simulink model "BLDC_model"  (R2020a)
settings: Solver=VariableStepAuto  StartTime=0.0  StopTime=10.0  RelTol=1e-3
InitFcn:
  | BLDC_FOC_Params
values from neighbouring files (symbols this model uses):
  AlignmentDuration = 3 * TimeConstant_s    (= 0.2025)    [BLDC_FOC_Params.m]
  AlignmentDuration_s = 1    [BLDC_FOC_Params.m]
  B = FrictionCoefficient_Nms    (= 1e-06)    [BLDC_FOC_Params.m]    (also in BldcModel.m = [1/Ls 0 0 0; systemDynamicsFunction.m = evalin('base','B'))
  J = RotorInertia_KgM2    (= 1.1e-07)    [BLDC_FOC_Params.m]    (also in systemDynamicsFunction.m = evalin('base','J'))
  Ke = BackEmfConstant_VRads    (= 0.00505253787593)    [BLDC_FOC_Params.m]    (also in systemDynamicsFunction.m = evalin('base','Ke'))
  Ls = PhaseSelfInductance_H    (= 0)    [BLDC_FOC_Params.m]    (also in systemDynamicsFunction.m = evalin('base','Ls'))
  MotorPolePairs = 4    [BLDC_FOC_Params.m]
  P = MotorPolePairs    (= 4)    [BLDC_FOC_Params.m]    (also in systemDynamicsFunction.m = evalin('base','P'))
  RampupDuration_s = 1    [BLDC_FOC_Params.m]
  Rs = PhaseResistance_Ohm    (= 0)    [BLDC_FOC_Params.m]    (also in systemDynamicsFunction.m = evalin('base','Rs'))
  Svpwm_freq_hz = 20000    [BLDC_FOC_Params.m]
  Ts = 0.0001    [BLDC_FOC_Params.m]
libraries: ee_lib x20, nesl_utility x10, BLDC_Dynamics_lib x6, fl_lib x5, eePwmGenerator x2, simulink x2, eeStairGenerator x1
settings Model: Creator=enzoe  LastModifiedBy=enzoe

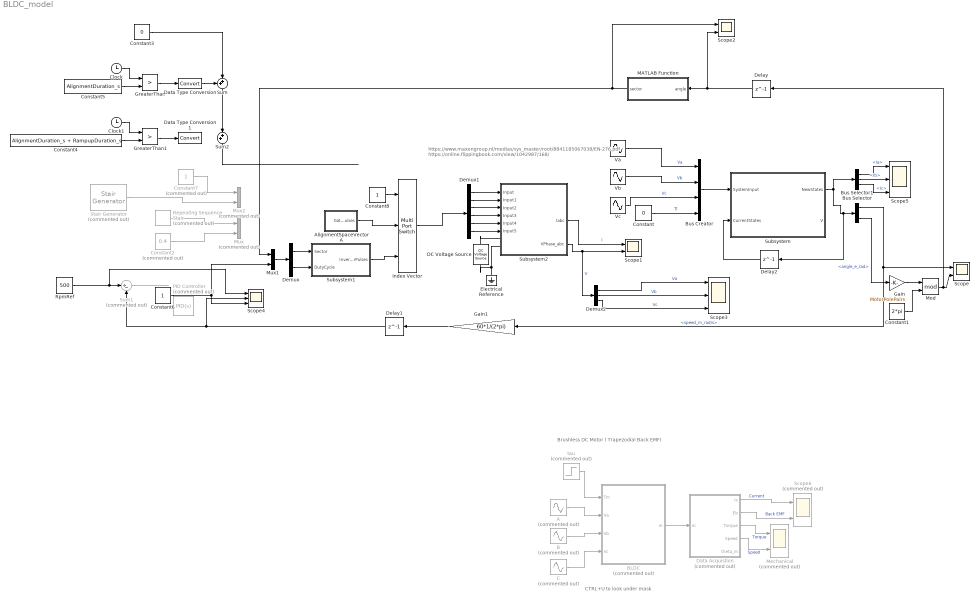
== system BLDC_model ==
  note: https://www.maxongroup.nl/medias/sys_master/root/8841185067038/EN-276.pdf
      | https://online.flippingbook.com/view/1042987/168/
  note: CTRL+U to look under mask
  note: Brushless DC Motor ( Trapezodial Back EMF)
  A : Sin  Commented=on  Amplitude=220*sqrt(2)  Frequency=2*pi*50  SampleTime=Ts
  AlignmentSpaceVectorA : Subsystem
  B : Sin  Commented=on  Amplitude=220*sqrt(2)  Frequency=2*pi*50  Phase=-2*pi/3  SampleTime=Ts
  BLDC : Subsystem  Commented=on  mask(Brushless DC Motor :){Rs=1.43, Ls=9.4e-3, flux=0.2158, J=1.5e-3, B=2e-3, p=4}
      mask prompts: Rs "Resistance - Rs [ohms] :"; Ls "Inductance - Ls [H] :"; flux "Flux - [wb]"; J "Rotor Inertia - J [kg-m^2]"; B "Friction Coefficient - B :"; p "No: poles of Motor :"
      mask help: Brushless DC Motor inducing trapezoidal Back EMF
      mask init:
      | trap=0.5;
      mask Display: fprintf('BLDC')
  Bus Creator : BusCreator  Inputs=4
  Bus Selector : BusSelector  OutputSignals=speed_m_rad/s,angle_e_rad
  Bus Selector1 : BusSelector  OutputSignals=Ia,Ib,Ic
  C : Sin  Commented=on  Amplitude=220*sqrt(2)  Frequency=2*pi*50  Phase=2*pi/3  SampleTime=Ts
  Clock : Clock
  Clock1 : Clock
  Constant : Constant  Value=0
  Constant1 : Constant  Value=2*pi
  Constant2 : Constant  Commented=on  Value=0.4
  Constant3 : Constant  Value=0
  Constant4 : Constant  Value=AlignmentDuration_s + RampupDuration_s
  Constant5 : Constant  Value=AlignmentDuration_s
  Constant6 : Constant
  Constant7 : Constant  Commented=on
  Constant8 : Constant
  DC Voltage Source : ee_lib/Additional Components/SPICE Sources/DC Voltage Source  DC=BatteryVoltage V
  Data Acquistion : Subsystem  Commented=on
  Data Type Conversion : DataTypeConversion
  Data Type Conversion1 : DataTypeConversion
  Delay : Delay  DelayLength=1
  Delay1 : Delay  DelayLength=1
  Delay2 : Delay  DelayLength=1
  Demux : Demux  Outputs=2
  Demux1 : Demux  Outputs=6
  Demux2 : Demux  Outputs=3
  Electrical Reference : fl_lib/Electrical/Electrical Elements/Electrical Reference
  Gain : Gain  Gain=MotorPolePairs
  Gain1 : Gain  Gain=60*1/(2*pi)
  GreaterThan : RelationalOperator  Operator=>  OutDataTypeStr=boolean  RndMeth=Simplest
  GreaterThan1 : RelationalOperator  Operator=>  OutDataTypeStr=boolean  RndMeth=Simplest
  Index Vector : MultiPortSwitch  DataPortOrder=Zero-based contiguous  Inputs=2  zeroidx=on
  MATLAB Function : MATLAB Function  TreatAsAtomicUnit=on
  Mechanical : Scope  Commented=on  NumInputPorts=2
  Mod : Math  Operator=mod  SaturateOnIntegerOverflow=on
  Mux : Mux  Commented=on  Inputs=2
  Mux1 : Mux  Inputs=2
  Mux2 : Mux  Commented=on  Inputs=2
  PID Controller : simulink/Continuous/PID Controller  Commented=on  Controller=PID  Form=Parallel  TimeDomain=Continuous-time  UseExternalTs=off  SampleTime=-1  IntegratorMethod=Forward Euler  FilterMethod=Forward Euler  ControllerParametersSource=internal  P=0.01  I=0.01  D=0  UseFilter=on  N=100  TunerSelectOption=Transfer Function Based (PID Tuner App)  InitialConditionSource=internal  InitialConditionForIntegrator=0  InitialConditionForFilter=0  DifferentiatorICPrevScaledInput=0  ExternalReset=none  TrackingMode=off  Kt=1  LimitOutput=off  UpperSaturationLimit=inf  LowerSaturationLimit=-inf  LinearizeAsGain=on  AntiWindupMode=none  Kb=1  POutMin=[]  POutMax=[]  IOutMin=[]  IOutMax=[]  DOutMin=[]  DOutMax=[]  NOutMin=[]  NOutMax=[]  SumOutMin=[]  SumOutMax=[]  SaturationOutMin=[]  SaturationOutMax=[]  PParamMin=[]  PParamMax=[]  IParamMin=[]  IParamMax=[]  DParamMin=[]  DParamMax=[]  NParamMin=[]  NParamMax=[]  KbParamMin=[]  KbParamMax=[]  KtParamMin=[]  KtParamMax=[]  KbOutMin=[]  KbOutMax=[]  KtOutMin=[]  KtOutMax=[]  IntegratorOutMin=[]  IntegratorOutMax=[]  FilterOutMin=[]  FilterOutMax=[]  SumI1OutMin=[]  SumI1OutMax=[]  SumI2OutMin=[]  SumI2OutMax=[]  SumI3OutMin=[]  SumI3OutMax=[]  SumI4OutMin=[]  SumI4OutMax=[]  SumDOutMin=[]  SumDOutMax=[]  DifferentiatorOutMin=[]  DifferentiatorOutMax=[]  FilterDiffOutCoefMin=[]  FilterDiffOutCoefMax=[]  ReciprocalOutMin=[]  ReciprocalOutMax=[]  SumDenOutMin=[]  SumDenOutMax=[]  SumNumOutMin=[]  SumNumOutMax=[]  DivideOutMin=[]  DivideOutMax=[]  UdiffTsProdOutMin=[]  UdiffTsProdOutMax=[]  NTsProdOutMin=[]  NTsProdOutMax=[]  UintegralTsProdOutMin=[]  UintegralTsProdOutMax=[]  UngainTsProdOutMin=[]  UngainTsProdOutMax=[]  IntegratorContinuousStateAttributes=''  IntegratorStateMustResolveToSignalObject=off  IntegratorRTWStateStorageClass=Auto  FilterContinuousStateAttributes=''  FilterStateMustResolveToSignalObject=off  FilterRTWStateStorageClass=Auto  ParallelPVariant=InternalParameters  IdealPVariant=Disabled  IVariant=InternalParameters  DVariant=InternalParameters  IntegratorVariant=Continuous  SatVariant=Disabled  AWVariant=Passthrough  PCopyVariant=Disabled  TRVariant=Disabled  FdbkBlocksVariant=Forward  IdealPFdbkVariant=Disabled  SatFdbkVariant=Disabled  DerivativeFilterVariant=ContFilter  NVariant=InternalParameters  NCopyVariant=Disabled  FilterICVariant=InternalICsFilter  IntegratorICVariant=InternalICs  ExternalResetVariant=Disabled  TRSumVariant=Passthrough  SumFdbkVariant=Disabled  SumVariant=Sum_PID  TsampFilterVariant=InternalTs  TsampNgainVariant=Passthrough  TsampIntegralVariant=Passthrough
  Repeating Sequence Stair : simulink/Sources/Repeating Sequence Stair  Commented=on  OutValues=[1 2 3 4 5 6].'  tsamp=0.01  OutMin=[]  OutMax=[]  OutDataTypeStr=double  OutputDataTypeScalingMode=double  OutDataType=fixdt(0,8)  ConRadixGroup=Best Precision: Vector-wise  OutScaling=2^-12
  RpmRef : Constant  Value=500
  Scope : Scope  NumInputPorts=2
  Scope1 : Scope  NumInputPorts=2
  Scope2 : Scope  NumInputPorts=2
  Scope3 : Scope  NumInputPorts=3
  Scope4 : Scope  NumInputPorts=3
  Scope5 : Scope  NumInputPorts=3
  Scope6 : Scope  Commented=on  NumInputPorts=2
  Stair Generator : eeStairGenerator/Stair Generator  Commented=on  LabelModeActiveChoice=Discrete  TimeInput=[0 AlignmentDuration/3 2*AlignmentDuration/3 AlignmentDuration]  AmplitudeInput=[0 0.2 0.3 0.4]  SampleTime=Ts  RepeatPattern=off  OutDataTypeStr=double
      settings: SourceProductBaseCode=PS
  Subsystem : Subsystem
  Subsystem1 : Subsystem
  Subsystem2 : Subsystem
      settings: PortSchema="{\"entries\":[{\"content\":{\"sides\":[{\"content\":{\"connectorIds\":[\"In1\",\"In2\",\"In3\",\"In4\",\"In5\",\"In6\",\"LConn1\",\"LConn2\"]},\"type\":\"ConnectorPlacement.EquallySpacedRectSide\",\"uuid\":\"4a91dc72-3770-4abf-bed3-c4a9f6b4b65e\"},{\"content\":{\"connectorIds\":[\"RConn1\",\"Out1\",\"Out2\"],\"side\":\"RIGHT\"},\"type\":\"ConnectorPlacement.EquallySpacedRectSide\",\"uuid\":\"c06ed33e-65a1-40a2-85db-2ae3e949e0d2\"},{\"content\":{\"connectorIds\":[],\"side\":\"TOP\"},\"type\":\"ConnectorPlacement.EquallySpacedRectSide\",\"uuid\":\"0b7af1c1-9cb6-4ccc-8dcc-bc330691322d\"}]},\"type\":\"ConnectorPlacement.EquallySpacedConnector\",\"uuid\":\"fc3d9dc5-347b-4e6e-ad3c-0830f77ecff8\"}],\"packageUris\":[\"http://schema.mathworks.com/mf0/Connector/19700101\"],\"version\":\"1.0\"}"
  Sum : Sum  Inputs=++|
  Sum1 : Sum  Commented=on  Inputs=|+-
  Sum2 : Sum  Inputs=++|
  Va : Sin  Amplitude=12*sqrt(2)  Frequency=2*pi*50  SampleTime=Ts
  Vb : Sin  Amplitude=12*sqrt(2)  Frequency=2*pi*50  Phase=-2*pi/3  SampleTime=Ts
  Vc : Sin  Amplitude=12*sqrt(2)  Frequency=2*pi*50  Phase=2*pi/3  SampleTime=Ts
  tau : Step  Commented=on  Time=0.5  After=10  SampleTime=0
  wires:
  Demux2/1 -> Scope3/1  "Va"
  Bus Creator/1 -> Subsystem/1(SystemInput)
  Constant/1 -> Bus Creator/4  "Tl"
  Demux2/3 -> Scope3/3  "Vc"
  Demux2/2 -> Scope3/2  "Vb"
  Delay2/1 -> Subsystem/2(CurrentStates)
  Subsystem1/1(InverterPulses) -> Index Vector/3
  AlignmentSpaceVectorA/1(GatePulses) -> Index Vector/2
  Gain1/1 -> Delay1/1
  Delay1/1 -> Scope4/2, Sum1/2
  Constant4/1 -> GreaterThan1/2
  Sum/1 -> Sum2/2
  GreaterThan1/1 -> Data Type Conversion1/1
  Demux/1 -> Subsystem1/1(Sector)
  Constant6/1 -> Mux1/2, Scope4/3
  RpmRef/1 -> Scope4/1, Sum1/1
  Index Vector/1 -> Demux1/1
  Demux1/1 -> Subsystem2/1(Input)
  Sum1/1 -> ?
  Clock1/1 -> GreaterThan1/1
  Stair Generator/1 -> Mux2/2
  Subsystem2/2(VPhase_abc) -> Scope1/2, Demux2/1  "V"
  Mux1/1 -> Demux/1
  Data Type Conversion/1 -> Sum/1
  Subsystem2/1(Iabc) -> Scope1/1  "I"
  Constant7/1 -> Mux2/1
  Constant5/1 -> GreaterThan/2
  Delay/1 -> Scope2/2, MATLAB Function/1(angle)
  Demux1/5 -> Subsystem2/5(Input4)
  Demux1/4 -> Subsystem2/4(Input3)
  Constant2/1 -> Mux/2
  Clock/1 -> GreaterThan/1
  Sum2/1 -> ?
  Repeating Sequence Stair/1 -> Mux/1
  Demux/2 -> Subsystem1/2(DutyCycle)
  Constant3/1 -> Sum/2
  Mod/1 -> Delay/1, Scope/2
  MATLAB Function/1(sector) -> Mux1/1, Scope2/1
  Demux1/6 -> Subsystem2/6(Input5)
  Demux1/2 -> Subsystem2/2(Input1)
  GreaterThan/1 -> Data Type Conversion/1
  Bus Selector/1 -> Gain1/1, Scope/1  "<speed_m_rad/s>"
  Demux1/3 -> Subsystem2/3(Input2)
  Constant1/1 -> Mod/2
  Subsystem/1(NewStates) -> Delay2/1, Bus Selector/1, Bus Selector1/1
  Bus Selector1/1 -> Scope5/1  "<Ia>"
  Bus Selector1/2 -> Scope5/2  "<Ib>"
  Bus Selector1/3 -> Scope5/3  "<Ic>"
  Constant8/1 -> Index Vector/1
  Data Acquistion/4(Speed) -> Mechanical/2  "Speed"
  tau/1 -> BLDC/1(Tm)
  Data Acquistion/2(Eb) -> Scope6/2  "Back EMF"
  Data Acquistion/3(Torque) -> Mechanical/1  "Torque"
  Data Acquistion/1(Is) -> Scope6/1  "Current"
  BLDC/1(m) -> Data Acquistion/1(m)
  A/1 -> BLDC/2(Va)
  B/1 -> BLDC/3(Vb)
  C/1 -> BLDC/4(Vc)
  Va/1 -> Bus Creator/1  "Va"
  Vb/1 -> Bus Creator/2  "Vb"
  Vc/1 -> Bus Creator/3  "Vc"
  Bus Selector/2 -> Gain/1  "<angle_e_rad>"
  Gain/1 -> Mod/1
  connections:
  Electrical Reference/LConn1 -- Subsystem2/LConn2 -- DC Voltage Source/RConn1
  DC Voltage Source/LConn1 -- Subsystem2/LConn1

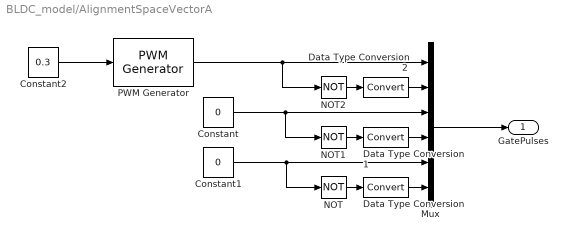
== system BLDC_model/AlignmentSpaceVectorA ==
  Constant : Constant  Value=0
  Constant1 : Constant  Value=0
  Constant2 : Constant  Value=0.3
  Data Type Conversion : DataTypeConversion
  Data Type Conversion1 : DataTypeConversion
  Data Type Conversion2 : DataTypeConversion
  Mux : Mux  Inputs=6
  NOT : Logic  Operator=NOT  IconShape=distinctive  AllPortsSameDT=off  OutDataTypeStr=boolean
  NOT1 : Logic  Operator=NOT  IconShape=distinctive  AllPortsSameDT=off  OutDataTypeStr=boolean
  NOT2 : Logic  Operator=NOT  IconShape=distinctive  AllPortsSameDT=off  OutDataTypeStr=boolean
  PWM Generator : eePwmGenerator/PWM Generator  CarrCount=Up  Tper=1/Svpwm_freq_hz  Ts=Ts
  GatePulses : Outport
  wires:
  Mux/1 -> GatePulses/1
  NOT1/1 -> Data Type Conversion1/1
  NOT2/1 -> Data Type Conversion2/1
  Constant1/1 -> Mux/5, NOT/1
  Constant/1 -> Mux/3, NOT1/1
  Constant2/1 -> PWM Generator/1
  PWM Generator/1 -> Mux/1, NOT2/1
  NOT/1 -> Data Type Conversion/1
  Data Type Conversion/1 -> Mux/6
  Data Type Conversion1/1 -> Mux/4
  Data Type Conversion2/1 -> Mux/2

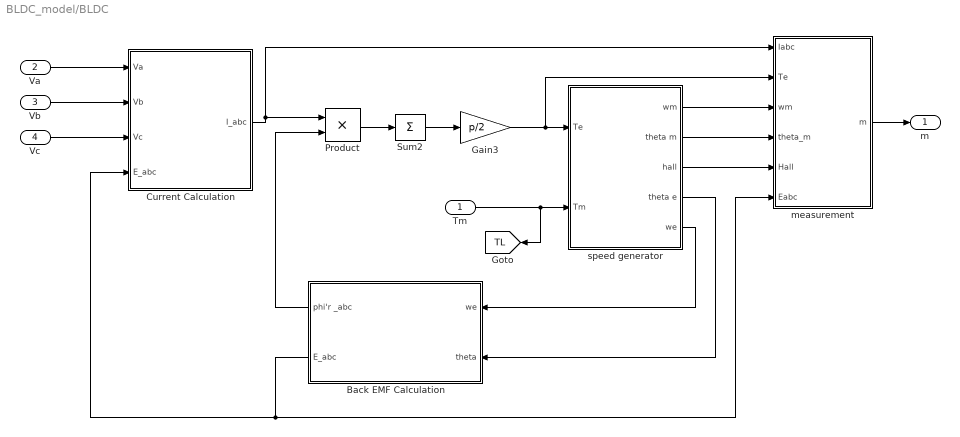
== system BLDC_model/BLDC ==
  Tm : Inport
  Va : Inport  Port=2
  Vb : Inport  Port=3
  Vc : Inport  Port=4
  Back EMF Calculation : Subsystem
  Current Calculation : Subsystem
  Gain3 : Gain  Gain=p/2  SaturateOnIntegerOverflow=on  OutDataTypeStr=Inherit: Same as input  ParamDataTypeStr=Inherit: Same as input
  Product : Product  SaturateOnIntegerOverflow=on  OutDataTypeStr=Inherit: Same as first input
  Sum2 : Sum  Inputs=+  SaturateOnIntegerOverflow=on
  measurement : Subsystem
  speed generator : Subsystem
  m : Outport
  tag scope: TL=global
  wires:
  Vc/1 -> Current Calculation/3(Vc)
  Vb/1 -> Current Calculation/2(Vb)
  Va/1 -> Current Calculation/1(Va)
  measurement/1(m) -> m/1
  speed generator/4(theta e) -> Back EMF Calculation/2(theta)
  speed generator/3(hall) -> measurement/5(Hall)
  speed generator/2(theta m) -> measurement/4(theta_m)
  speed generator/1(wm) -> measurement/3(wm)
  Tm/1 -> [TL], speed generator/2(Tm)
  Back EMF Calculation/1(phi'r _abc) -> Product/2
  Product/1 -> Sum2/1
  Sum2/1 -> Gain3/1
  Gain3/1 -> measurement/2(Te), speed generator/1(Te)
  speed generator/5(we) -> Back EMF Calculation/1(we)
  Back EMF Calculation/2(E_abc) -> Current Calculation/4(E_abc), measurement/6(Eabc)
  Current Calculation/1(I_abc) -> measurement/1(Iabc), Product/1

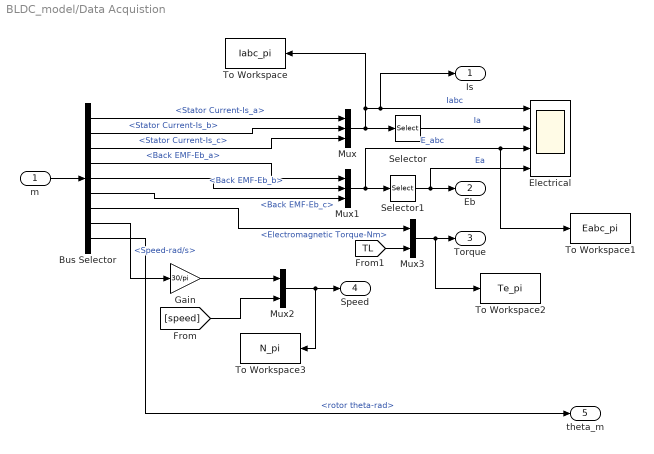
== system BLDC_model/Data Acquistion ==
  m : Inport
  Bus Selector : BusSelector  OutputSignals=Stator Current-Is_a,Stator Current-Is_b,Stator Current-Is_c,Back EMF-Eb_a,Back EMF-Eb_b,Back EMF-Eb_c,Electromagnetic Torque-Nm,Speed-rad/s,rotor theta-rad
  Electrical : Scope  NumInputPorts=4
  Gain : Gain  Gain=30/pi
  Mux : Mux  Inputs=3
  Mux1 : Mux  Inputs=3
  Mux2 : Mux  Inputs=2
  Mux3 : Mux  Inputs=2
  Selector : Selector  InputPortWidth=3  IndexOptions=Index vector (dialog)  Indices=[1 ]  OutputSizes=1
  Selector1 : Selector  InputPortWidth=3  IndexOptions=Index vector (dialog)  Indices=[1 ]  OutputSizes=1
  To Workspace : ToWorkspace  VariableName=Iabc_pi  SampleTime=Ts
  To Workspace1 : ToWorkspace  VariableName=Eabc_pi  SampleTime=Ts
  To Workspace2 : ToWorkspace  VariableName=Te_pi  SampleTime=Ts
  To Workspace3 : ToWorkspace  VariableName=N_pi  SampleTime=Ts
  Is : Outport
  Eb : Outport  Port=2
  Torque : Outport  Port=3
  Speed : Outport  Port=4
  theta_m : Outport  Port=5
  wires:
  Mux3/1 -> To Workspace2/1, Torque/1
  [TL] -> Mux3/2
  [speed] -> Mux2/2
  Mux2/1 -> To Workspace3/1, Speed/1
  Gain/1 -> Mux2/1
  Selector1/1 -> Electrical/4, Eb/1  "Ea"
  Selector/1 -> Electrical/2  "Ia"
  Bus Selector/8 -> Gain/1  "<Speed-rad/s>"
  Bus Selector/7 -> Mux3/1  "<Electromagnetic Torque-Nm>"
  Mux1/1 -> To Workspace1/1, Electrical/3, Selector1/1  "E_abc"
  Bus Selector/6 -> Mux1/3  "<Back EMF-Eb_c>"
  Bus Selector/5 -> Mux1/2  "<Back EMF-Eb_b>"
  Bus Selector/4 -> Mux1/1  "<Back EMF-Eb_a>"
  Mux/1 -> Is/1, Electrical/1, To Workspace/1, Selector/1  "Iabc"
  Bus Selector/3 -> Mux/3  "<Stator Current-Is_c>"
  Bus Selector/2 -> Mux/2  "<Stator Current-Is_b>"
  Bus Selector/1 -> Mux/1  "<Stator Current-Is_a>"
  m/1 -> Bus Selector/1
  Bus Selector/9 -> theta_m/1  "<rotor theta-rad>"

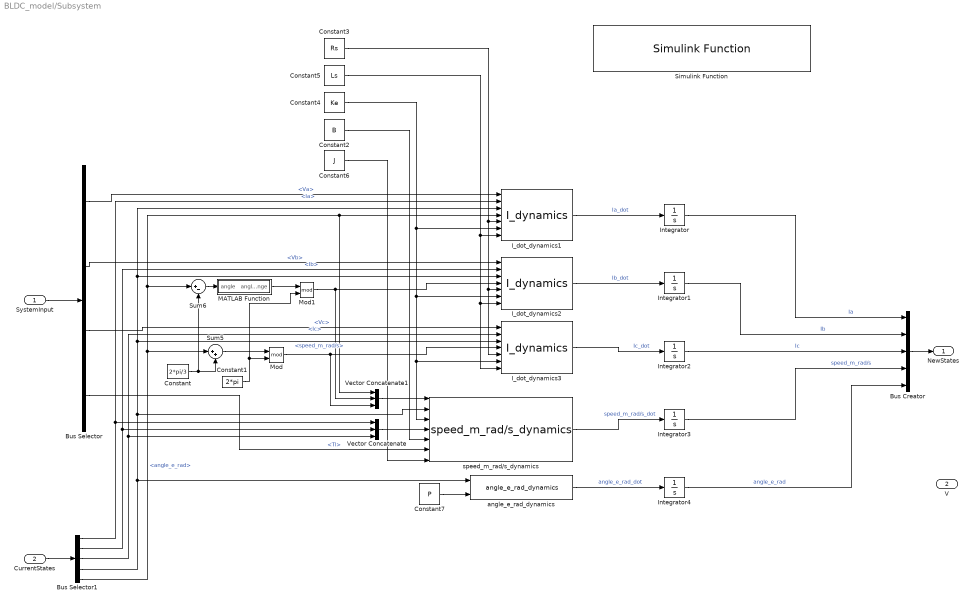
== system BLDC_model/Subsystem ==
  SystemInput : Inport
  CurrentStates : Inport  Port=2
  Bus Creator : BusCreator  Inputs=5
  Bus Selector : BusSelector  OutputSignals=Va,Vb,Vc,Tl
  Bus Selector1 : BusSelector  OutputSignals=Ia,Ib,Ic,speed_m_rad/s,angle_e_rad
  Constant : Constant  Value=2*pi/3
  Constant1 : Constant  Value=2*pi
  Constant2 : Constant  Value=B
  Constant3 : Constant  Value=Rs
  Constant4 : Constant  Value=Ke
  Constant5 : Constant  Value=Ls
  Constant6 : Constant  Value=J
  Constant7 : Constant  Value=P
  I_dot_dynamics1 : BLDC_Dynamics_lib/I_dynamics  SystemSampleTime=-1  Latency=0  AutoFrameSizeCalculation=off
  I_dot_dynamics2 : BLDC_Dynamics_lib/I_dynamics  SystemSampleTime=-1  Latency=0  AutoFrameSizeCalculation=off
  I_dot_dynamics3 : BLDC_Dynamics_lib/I_dynamics  SystemSampleTime=-1  Latency=0  AutoFrameSizeCalculation=off
  Integrator{,1..4} (5 alike) : Integrator
  MATLAB Function : MATLAB Function  TreatAsAtomicUnit=on
  Mod : Math  Operator=mod  SaturateOnIntegerOverflow=on
  Mod1 : Math  Operator=mod  SaturateOnIntegerOverflow=on
  Simulink Function : BLDC_Dynamics_lib/Simulink Function  SystemSampleTime=-1  Latency=0  AutoFrameSizeCalculation=off
  Sum5 : Sum  Inputs=|++
  Sum6 : Sum  Inputs=|+-
  Vector Concatenate : Concatenate  NumInputs=3
  Vector Concatenate1 : Concatenate  NumInputs=3
  angle_e_rad_dynamics : BLDC_Dynamics_lib/angle_e_rad_dynamics  SystemSampleTime=-1  Latency=0  AutoFrameSizeCalculation=off
  speed_m_rad/s_dynamics : BLDC_Dynamics_lib/speed_m_rad//s_dynamics  SystemSampleTime=-1  Latency=0  AutoFrameSizeCalculation=off
  NewStates : Outport
  V : Outport  Port=2
  wires:
  Bus Creator/1 -> NewStates/1
  Integrator/1 -> Bus Creator/1  "Ia"
  Integrator1/1 -> Bus Creator/2  "Ib"
  Integrator2/1 -> Bus Creator/3  "Ic"
  Integrator3/1 -> Bus Creator/4  "speed_m_rad/s"
  Integrator4/1 -> Bus Creator/5  "angle_e_rad"
  SystemInput/1 -> Bus Selector/1
  CurrentStates/1 -> Bus Selector1/1
  Bus Selector1/1 -> I_dot_dynamics1/2, Vector Concatenate/1  "<Ia>"
  Bus Selector1/2 -> I_dot_dynamics2/2, Vector Concatenate/2  "<Ib>"
  Bus Selector1/3 -> I_dot_dynamics3/2, Vector Concatenate/3  "<Ic>"
  Bus Selector1/4 -> angle_e_rad_dynamics/1, I_dot_dynamics3/3, I_dot_dynamics2/3, I_dot_dynamics1/3, speed_m_rad/s_dynamics/2  "<speed_m_rad/s>"
  Bus Selector1/5 -> Vector Concatenate1/1, I_dot_dynamics1/4, Sum6/1, Sum5/1  "<angle_e_rad>"
  I_dot_dynamics3/1 -> Integrator2/1  "Ic_dot"
  angle_e_rad_dynamics/1 -> Integrator4/1  "angle_e_rad_dot"
  I_dot_dynamics1/1 -> Integrator/1  "Ia_dot"
  Bus Selector/1 -> I_dot_dynamics1/1  "<Va>"
  Bus Selector/2 -> I_dot_dynamics2/1  "<Vb>"
  Bus Selector/4 -> speed_m_rad/s_dynamics/6  "<Tl>"
  I_dot_dynamics2/1 -> Integrator1/1  "Ib_dot"
  Constant/1 -> Sum6/2, Sum5/2
  Constant1/1 -> Mod1/2, Mod/2
  Sum5/1 -> Mod/1
  Constant3/1 -> I_dot_dynamics1/5, I_dot_dynamics3/5, I_dot_dynamics2/5
  Constant4/1 -> I_dot_dynamics1/6, I_dot_dynamics2/6, I_dot_dynamics3/6, speed_m_rad/s_dynamics/3
  Constant5/1 -> I_dot_dynamics3/7, I_dot_dynamics2/7, I_dot_dynamics1/7
  Mod1/1 -> Vector Concatenate1/2, I_dot_dynamics2/4
  Bus Selector/3 -> I_dot_dynamics3/1  "<Vc>"
  Mod/1 -> Vector Concatenate1/3, I_dot_dynamics3/4
  Vector Concatenate/1 -> speed_m_rad/s_dynamics/4
  Vector Concatenate1/1 -> speed_m_rad/s_dynamics/1
  Constant2/1 -> speed_m_rad/s_dynamics/5
  Constant6/1 -> speed_m_rad/s_dynamics/7
  speed_m_rad/s_dynamics/1 -> Integrator3/1  "speed_m_rad/s_dot"
  Constant7/1 -> angle_e_rad_dynamics/2
  Sum6/1 -> MATLAB Function/1(angle)
  MATLAB Function/1(angle_in_range) -> Mod1/1

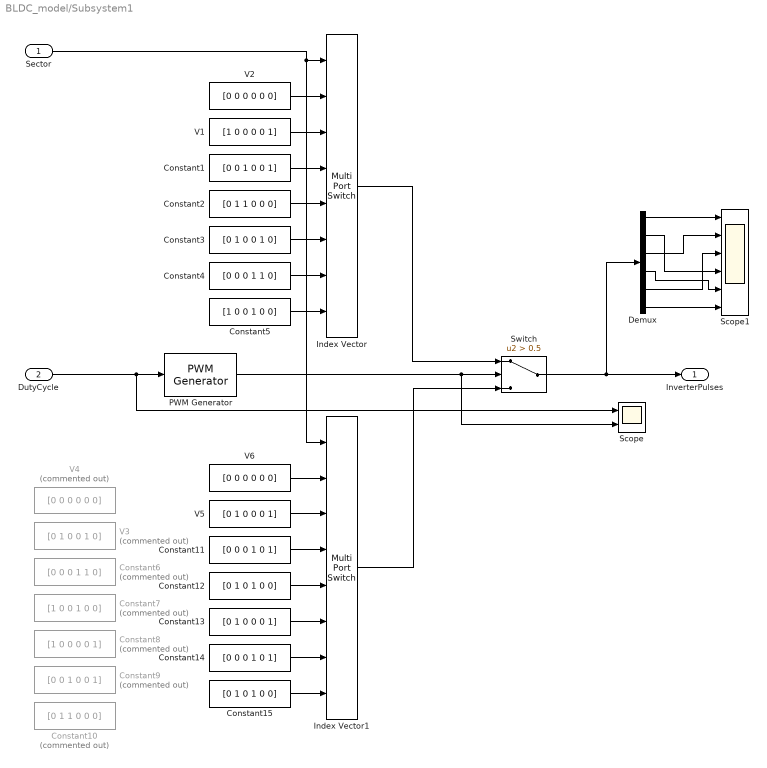
== system BLDC_model/Subsystem1 ==
  Sector : Inport
  DutyCycle : Inport  Port=2
  Constant1 : Constant  Value=[0 0 1 0 0 1]
  Constant10 : Constant  Commented=on  Value=[0 1 1 0 0 0]
  Constant11 : Constant  Value=[0 0 0 1 0 1]
  Constant12 : Constant  Value=[0 1 0 1 0 0]
  Constant13 : Constant  Value=[0 1 0 0 0 1]
  Constant14 : Constant  Value=[0 0 0 1 0 1]
  Constant15 : Constant  Value=[0 1 0 1 0 0]
  Constant2 : Constant  Value=[0 1 1 0 0 0]
  Constant3 : Constant  Value=[0 1 0 0 1 0]
  Constant4 : Constant  Value=[0 0 0 1 1 0]
  Constant5 : Constant  Value=[1 0 0 1 0 0]
  Constant6 : Constant  Commented=on  Value=[0 0 0 1 1 0]
  Constant7 : Constant  Commented=on  Value=[1 0 0 1 0 0]
  Constant8 : Constant  Commented=on  Value=[1 0 0 0 0 1]
  Constant9 : Constant  Commented=on  Value=[0 0 1 0 0 1]
  Demux : Demux  Outputs=6
  Index Vector : MultiPortSwitch  DataPortOrder=Zero-based contiguous  Inputs=7  zeroidx=on
  Index Vector1 : MultiPortSwitch  DataPortOrder=Zero-based contiguous  Inputs=7  zeroidx=on
  PWM Generator : eePwmGenerator/PWM Generator  CarrCount=Up  Tper=1/Svpwm_freq_hz  Ts=Ts
  Scope : Scope  NumInputPorts=2
  Scope1 : Scope  NumInputPorts=6
  Switch : Switch  Criteria=u2 > Threshold  Threshold=0.5
  V1 : Constant  Value=[1 0 0 0 0 1]
  V2 : Constant  Value=[0 0 0 0 0 0]
  V3 : Constant  Commented=on  Value=[0 1 0 0 1 0]
  V4 : Constant  Commented=on  Value=[0 0 0 0 0 0]
  V5 : Constant  Value=[0 1 0 0 0 1]
  V6 : Constant  Value=[0 0 0 0 0 0]
  InverterPulses : Outport
  wires:
  V1/1 -> Index Vector/3
  Constant1/1 -> Index Vector/4
  Constant2/1 -> Index Vector/5
  Constant3/1 -> Index Vector/6
  Constant4/1 -> Index Vector/7
  Constant5/1 -> Index Vector/8
  Index Vector/1 -> Switch/1
  Sector/1 -> Index Vector1/1, Index Vector/1
  V2/1 -> Index Vector/2
  DutyCycle/1 -> Scope/1, PWM Generator/1
  PWM Generator/1 -> Scope/2, Switch/2
  Constant12/1 -> Index Vector1/5
  Constant14/1 -> Index Vector1/7
  Constant13/1 -> Index Vector1/6
  Constant11/1 -> Index Vector1/4
  Constant15/1 -> Index Vector1/8
  V6/1 -> Index Vector1/2
  V5/1 -> Index Vector1/3
  Index Vector1/1 -> Switch/3
  Switch/1 -> Demux/1, InverterPulses/1
  Demux/1 -> Scope1/1
  Demux/3 -> Scope1/2
  Demux/5 -> Scope1/3
  Demux/2 -> Scope1/4
  Demux/4 -> Scope1/5
  Demux/6 -> Scope1/6

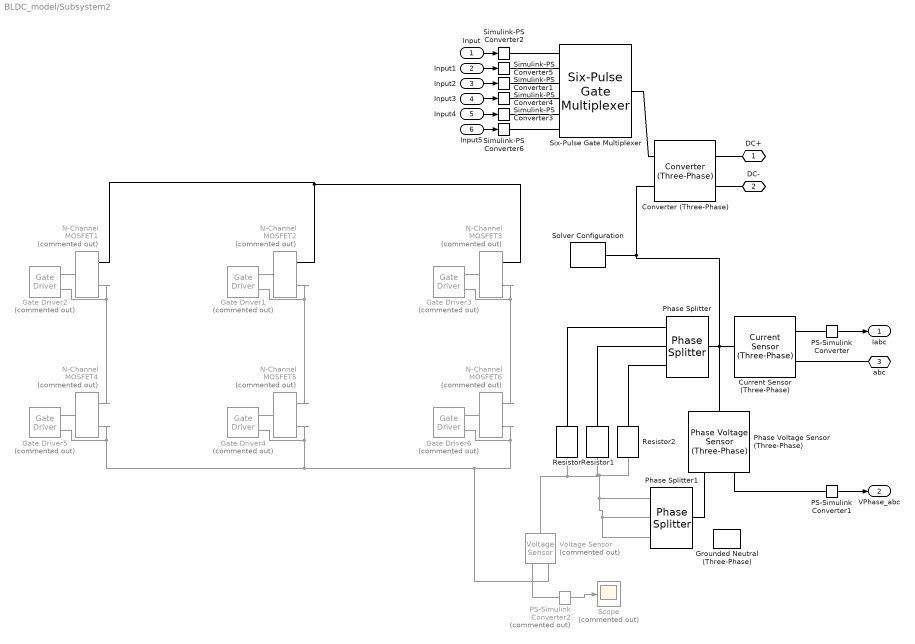
== system BLDC_model/Subsystem2 ==
  Input : Inport
  Input1 : Inport  Port=2
  Input2 : Inport  Port=3
  Input3 : Inport  Port=4
  Input4 : Inport  Port=5
  Input5 : Inport  Port=6
  Converter (Three-Phase) : ee_lib/Semiconductors & Converters/Converters/Converter (Three-Phase)  device_type=ee.enum.converters.switchingdevice.ideal  Vf=0.8 V  Ron=0.001 Ohm  Rds=0.001 Ohm  Goff=1e-6 1/Ohm  Vth=0.5 V  Vgt=1 V  Vgt_off=-1 V  Ih=1 A  diode_param=ee.enum.converters.protectiondiode.nodynamics  diode_Vf=0.8 V  diode_Ron=0.001 Ohm  diode_Goff=1e-5 1/Ohm  diode_C=50 nF  diode_iRM=-235 A  diode_iF=300 A  diode_idot=-50 A/us  diode_trr_param=ee.enum.converters.diodetrr.trr_factor  diode_trr_factor=3  diode_trr=15 us  diode_Qrr=1500 s*uA  snubber_type=ee.enum.converters.snubber.exclude  Rs=0.1 Ohm  Cs=1e-7 F
      settings: SourceProductBaseCode=PS
  Current Sensor (Three-Phase) : ee_lib/Sensors & Transducers/Current Sensor (Three-Phase)
  Gate Driver{1..6} (6 alike) : ee_lib/Semiconductors & Converters/Gate Driver  Commented=on  vHigh=15 V  vLow=0 V  parameterization=1  rHigh=2 Ohm  rLow=2 Ohm  tRise=20 ns  tFall=20 ns  cLoad=10 nF  enable_faults=0  t_fault=1 s  fault_type=1  uHighValue=0.7  uLowValue=0.3  tHigh=50 ns  tLow=50 ns  ZonTime_specify=off  ZonTime_priority=None  ZonTime=0 s  ZoffTime_specify=off  ZoffTime_priority=None  ZoffTime=0 s  uHigh=2.0 V  uLow=0.8 V
      settings: SourceProductBaseCode=PS  InternalSimscapePortConfiguration="{\"Bottom\":[],\"Left\":[{\"id\":\"u\",\"label\":\"u\",\"type\":\"input\"}],\"Right\":[{\"id\":\"G\",\"label\":\"G\",\"type\":\"foundation.electrical.electrical\"},{\"id\":\"S\",\"label\":\"S\",\"type\":\"foundation.electrical.electrical\"}],\"Top\":[]}"
  Grounded Neutral (Three-Phase) : ee_lib/Connectors & References/Grounded Neutral (Three-Phase)
      settings: SourceProductBaseCode=PS
  N-Channel MOSFET{1..6} (6 alike) : ee_lib/Semiconductors & Converters/N-Channel MOSFET  Commented=on  paramTerminal=ee.enum.mosfet.numberOfTerminals.three  parameterization=ee.enum.parameterization.datasheet  prmDatasheet=ee.enum.temperatureParameterization.none  prmEquCoeff=ee.enum.temperatureParameterization.none  Beta=5.0 A/V^2  Rds=0.025 Ohm  Id=6.0 A  Vgs=10 V  Vth=1.7 V  Vth0=1.7 V  lam=0 1/V  gamma_vth=0.5 V^0.50000  phib=0.5 V  Vth1=1.9071 V  Vbs1=-1 V  Vth2=2.066 V  Vbs2=-2 V  Tmeas=25 degC  RS=0.0001 Ohm  RD=0.01 Ohm  RB=0.001 Ohm  C_param=ee.enum.mosfet.capacitanceParam.fixedciss  C_GS=270 pF  C_GD=80 pF  C_DS=0 pF  C_iss=350 pF  C_rss=80 pF  C_oss=0 pF  charge_linearity_param=ee.enum.mosfet.cgdLinearity.constant  C_OX=200 pF  V_C_OX=-0.5 V  C_iss_vec=[720, 700, 590, 470, 390, 310] pF  C_rss_vec=[450, 400, 300, 190, 95, 55] pF  C_oss_vec=[900, 810, 690, 420, 270, 170] pF  C_GS_vec=[270, 300, 290, 280, 295, 255] pF  C_GD_vec=[450, 400, 300, 190, 95, 55] pF  C_DS_vec=[450, 410, 390, 230, 175, 115] pF  C_Vds_vec=[.1, .3, 1, 3, 10, 30] V  V_GS_for_cap_data=0 V  charge_linearity_param_vgb=ee.enum.mosfet.cgbLinearity.instantly  IsDiode=0 A  Vbi=0.6 V  n=1  Cj0Diode=0 pF  TT=50e-9 s  dVth_dT=-6 mV/K  dVth0_dT=-6 mV/K  Rds_T2=0.037 Ohm  Tmeas2=125 degC  BEXDatasheet=-1.5  BEXEquCoeff=-1.5  etaisDatasheet=3  etaisEquCoeff=3  TdeviceDatasheet=25 degC  TdeviceEquCoeff=25 degC  thermal_network_parameterization=ee.enum.thermalNetworkTopology.cauer  Rth=[0, 10] K/W  Rth_Foster=[4, 6] K/W  thermal_mass_parameterization=ee.enum.thermalNetwork.timeconstant  thermal_mass=[0, 1] J/K  thermal_mass_Foster=[1.5, 3] J/K  thermal_time_constant=[0, 10] s  thermal_time_constant_Foster=[6, 18] s  thermal_mass_initial_temperatures=[25, 25] degC  betaref=18 A/V^2  Vfbref=-1.1 V  gamma=3.5 V^0.50000  phib2ref=1 V  thesatref=0.4 1/V  alpha=0  Vp=5e-2 V  thesrref=0 1/V  m=8  Tref=25 degC  Cox=1500 pF  Cgso=100 pF  Cgdo=14 pF  Rsref=2e-3 Ohm  Rdref=0.17 Ohm  Rgref=8.4 Ohm  Rbref=2e-3 Ohm  Isref=5.2e-13 A  Cj0=480 pF  Tprm=1  etabet=1.3  Stvfb=5e-4 V/K  Stphib=-8.5e-4 V/K  etasat=1.04  etasr=0.65  etar=0.95  etais=3  Tsim=25 degC  T0=[25, 25] degC
  PS-Simulink Converter : nesl_utility/PS-Simulink Converter  PhysicalDomain=network_engine_domain  SubClassName=ps_output  LeftPortType=input  RightPortType=output  PseudoPeriodic=off  Frequencies=[]  Unit=inherit  AffineConversion=off
  PS-Simulink Converter1 : nesl_utility/PS-Simulink Converter  PhysicalDomain=network_engine_domain  SubClassName=ps_output  LeftPortType=input  RightPortType=output  PseudoPeriodic=off  Frequencies=[]  Unit=inherit  AffineConversion=off
  PS-Simulink Converter2 : nesl_utility/PS-Simulink Converter  Commented=on  PhysicalDomain=network_engine_domain  SubClassName=ps_output  LeftPortType=input  RightPortType=output  PseudoPeriodic=off  Frequencies=[]  Unit=inherit  AffineConversion=off
  Phase Splitter : ee_lib/Connectors & References/Phase Splitter
      settings: SourceProductBaseCode=PS
  Phase Splitter1 : ee_lib/Connectors & References/Phase Splitter
      settings: SourceProductBaseCode=PS
  Phase Voltage Sensor (Three-Phase) : ee_lib/Sensors & Transducers/Phase Voltage Sensor (Three-Phase)
      settings: SourceProductBaseCode=PS
  Resistor : fl_lib/Electrical/Electrical Elements/Resistor  R=1000 Ohm  i_specify=off  i_priority=None  i=0 A  i_nominal_specify=off  i_nominal_unit=A  i_nominal_value=1  v_specify=off  v_priority=None  v=0 V  v_nominal_specify=off  v_nominal_unit=V  v_nominal_value=1
  Resistor1 : fl_lib/Electrical/Electrical Elements/Resistor  R=1000 Ohm  i_specify=off  i_priority=None  i=0 A  i_nominal_specify=off  i_nominal_unit=A  i_nominal_value=1  v_specify=off  v_priority=None  v=0 V  v_nominal_specify=off  v_nominal_unit=V  v_nominal_value=1
  Resistor2 : fl_lib/Electrical/Electrical Elements/Resistor  R=1000 Ohm  i_specify=off  i_priority=None  i=0 A  i_nominal_specify=off  i_nominal_unit=A  i_nominal_value=1  v_specify=off  v_priority=None  v=0 V  v_nominal_specify=off  v_nominal_unit=V  v_nominal_value=1
  Scope : Scope  Commented=on
  Simulink-PS Converter{1..6} (6 alike) : nesl_utility/Simulink-PS Converter  PhysicalDomain=network_engine_domain  SubClassName=ps_input  LeftPortType=input  RightPortType=output  PseudoPeriodic=off  Frequencies=[]  NoiseDistribution=none  NoiseParameters=[]  Unit=1  AffineConversion=off  FilteringAndDerivatives=provide  SimscapeFilterOrder=1  InputFilterTimeConstant=0.001  UdotUserProvided=0
  Six-Pulse Gate Multiplexer : ee_lib/Semiconductors & Converters/Converters/Six-Pulse Gate Multiplexer  R=0 Ohm
      settings: SourceProductBaseCode=PS  InternalSimscapePortConfiguration="{\"Bottom\":[],\"Left\":[{\"id\":\"GaH\",\"label\":\"Ga(H)\",\"type\":\"input\"},{\"id\":\"GaL\",\"label\":\"Ga(L)\",\"type\":\"input\"},{\"id\":\"GbH\",\"label\":\"Gb(H)\",\"type\":\"input\"},{\"id\":\"GbL\",\"label\":\"Gb(L)\",\"type\":\"input\"},{\"id\":\"GcH\",\"label\":\"Gc(H)\",\"type\":\"input\"},{\"id\":\"GcL\",\"label\":\"Gc(L)\",\"type\":\"input\"}],\"Right\":[{\"id\":\"p\",\"label\":\"G\",\"type\":\"foundation.electrical.twelve_phase\"}],\"Top\":[]}"
  Solver Configuration : nesl_utility/Solver Configuration  PhysicalDomain=network_engine_domain  SubClassName=solver  LeftPortType=input  RightPortType=generic  Tones=[]  Harmonics=[]  SimulateNoise=off  Profile=off  UseLocalSampling=off  EnableSwitchedLinearOptims=on  FrequencyDomain=off  UseCCode=off  RelTol=0.001  AbsTol=1e-06  MinStep=1e-09  ToWorkspace=off  RevertToSquareIcSolve=off  NumHomotopyIterations=100  PhasorMode=off  PhasorModeNumHarmonics=1  DoDC=off  ResidualTolerance=1e-09  UseLocalSolver=on  LocalSolverChoice=NE_BACKWARD_EULER_ADVANCER  LocalSolverSampleTime=2e-5  DoFixedCost=on  MaxNonlinIter=4  MaxModeIter=2  LinearAlgebra=auto  EquationFormulation=NE_TIME_EF  DelaysMemoryBudget=1024  AutomaticFiltering=off  FilteringTimeConstant=0.001  PartitionStorageMethod=AS_NEEDED  PartitionMemoryBudget=1024  PartitionMethod=ROBUST
  Voltage Sensor : fl_lib/Electrical/Electrical Sensors/Voltage Sensor  Commented=on
  DC+ : PMIOPort  Side=Left
  DC- : PMIOPort  Port=2  Side=Left
  abc : PMIOPort  Port=3  Side=Right
  Iabc : Outport
  VPhase_abc : Outport  Port=2
  wires:
  Input/1 -> Simulink-PS Converter2/1
  Input1/1 -> Simulink-PS Converter5/1
  Input2/1 -> Simulink-PS Converter1/1
  Input3/1 -> Simulink-PS Converter4/1
  Input4/1 -> Simulink-PS Converter3/1
  Input5/1 -> Simulink-PS Converter6/1
  PS-Simulink Converter/1 -> Iabc/1
  PS-Simulink Converter1/1 -> VPhase_abc/1
  PS-Simulink Converter2/1 -> Scope/1
  connections:
  N-Channel MOSFET1/LConn1 -- Gate Driver2/RConn1
  N-Channel MOSFET4/RConn1 -- N-Channel MOSFET1/RConn2 -- Gate Driver2/RConn2
  Phase Splitter/RConn2 -- Resistor1/LConn1
  N-Channel MOSFET2/LConn1 -- Gate Driver1/RConn1
  N-Channel MOSFET3/LConn1 -- Gate Driver3/RConn1
  N-Channel MOSFET6/RConn1 -- N-Channel MOSFET3/RConn2 -- Gate Driver3/RConn2
  N-Channel MOSFET6/LConn1 -- Gate Driver6/RConn1
  N-Channel MOSFET4/RConn2 -- Voltage Sensor/RConn2 -- N-Channel MOSFET6/RConn2 -- Gate Driver6/RConn2 -- N-Channel MOSFET5/RConn2 -- Gate Driver4/RConn2 -- Gate Driver5/RConn2
  N-Channel MOSFET5/LConn1 -- Gate Driver4/RConn1
  N-Channel MOSFET4/LConn1 -- Gate Driver5/RConn1
  N-Channel MOSFET1/RConn1 -- N-Channel MOSFET3/RConn1 -- N-Channel MOSFET2/RConn1
  Current Sensor (Three-Phase)/RConn2 -- abc/RConn1
  Phase Voltage Sensor (Three-Phase)/LConn1 -- Converter (Three-Phase)/LConn2 -- Solver Configuration/RConn1 -- Phase Splitter/LConn1 -- Current Sensor (Three-Phase)/LConn1
  PS-Simulink Converter/LConn1 -- Current Sensor (Three-Phase)/RConn1
  PS-Simulink Converter1/LConn1 -- Phase Voltage Sensor (Three-Phase)/RConn1
  Voltage Sensor/LConn1 -- Resistor/RConn1 -- Phase Splitter1/RConn3 -- Phase Splitter1/RConn2 -- Phase Splitter1/RConn1 -- Resistor2/RConn1 -- Resistor1/RConn1
  PS-Simulink Converter2/LConn1 -- Voltage Sensor/RConn1
  DC+/RConn1 -- Converter (Three-Phase)/RConn1
  DC-/RConn1 -- Converter (Three-Phase)/RConn2
  Simulink-PS Converter2/RConn1 -- Six-Pulse Gate Multiplexer/LConn1
  Simulink-PS Converter5/RConn1 -- Six-Pulse Gate Multiplexer/LConn2
  Simulink-PS Converter1/RConn1 -- Six-Pulse Gate Multiplexer/LConn3
  Simulink-PS Converter4/RConn1 -- Six-Pulse Gate Multiplexer/LConn4
  Simulink-PS Converter3/RConn1 -- Six-Pulse Gate Multiplexer/LConn5
  Simulink-PS Converter6/RConn1 -- Six-Pulse Gate Multiplexer/LConn6
  Six-Pulse Gate Multiplexer/RConn1 -- Converter (Three-Phase)/LConn1
  Resistor/LConn1 -- Phase Splitter/RConn1
  N-Channel MOSFET2/RConn2 -- N-Channel MOSFET5/RConn1 -- Gate Driver1/RConn2
  Phase Splitter/RConn3 -- Resistor2/LConn1
  Phase Splitter1/LConn1 -- Phase Voltage Sensor (Three-Phase)/RConn2

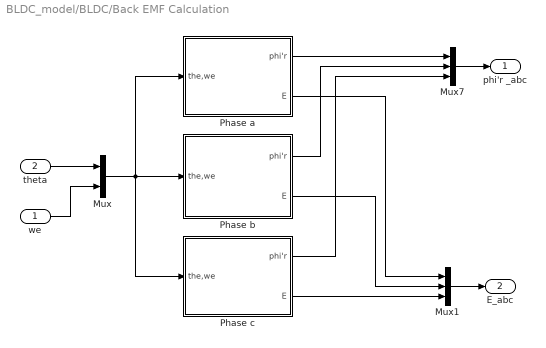
== system BLDC_model/BLDC/Back EMF Calculation ==
  we : Inport
  theta : Inport  Port=2
  Mux : Mux  Inputs=2
  Mux1 : Mux  Inputs=3
  Mux7 : Mux  Inputs=3
  Phase a : Subsystem
  Phase b : Subsystem
  Phase c : Subsystem
  phi'r _abc : Outport
  E_abc : Outport  Port=2
  wires:
  Mux1/1 -> E_abc/1
  Phase c/2(E) -> Mux1/3
  Phase b/2(E) -> Mux1/2
  Phase a/2(E) -> Mux1/1
  we/1 -> Mux/2
  theta/1 -> Mux/1
  Mux/1 -> Phase c/1(the,we), Phase b/1(the,we), Phase a/1(the,we)
  Phase a/1(phi'r) -> Mux7/1
  Phase b/1(phi'r) -> Mux7/2
  Phase c/1(phi'r) -> Mux7/3
  Mux7/1 -> phi'r _abc/1

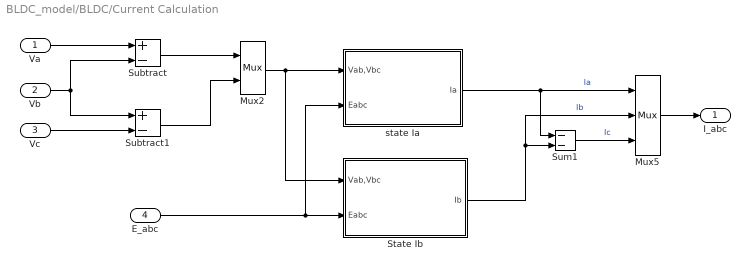
== system BLDC_model/BLDC/Current Calculation ==
  Va : Inport
  Vb : Inport  Port=2
  Vc : Inport  Port=3
  E_abc : Inport  Port=4
  Mux2 : Mux  Inputs=2
      settings: DisplayOption=signals
  Mux5 : Mux  Inputs=3
      settings: DisplayOption=signals
  State Ib : Subsystem
  Subtract : Sum  Inputs=+-
  Subtract1 : Sum  Inputs=+-
  Sum1 : Sum  Inputs=--  SaturateOnIntegerOverflow=on
  state Ia : Subsystem
  I_abc : Outport
  wires:
  State Ib/1(Ib) -> Sum1/2, Mux5/2  "Ib"
  Subtract1/1 -> Mux2/2
  Subtract/1 -> Mux2/1
  Vc/1 -> Subtract1/2
  Vb/1 -> Subtract1/1, Subtract/2
  Va/1 -> Subtract/1
  state Ia/1(Ia) -> Mux5/1, Sum1/1  "Ia"
  Sum1/1 -> Mux5/3  "Ic"
  Mux5/1 -> I_abc/1
  Mux2/1 -> State Ib/1(Vab,Vbc), state Ia/1(Vab,Vbc)
  E_abc/1 -> State Ib/2(Eabc), state Ia/2(Eabc)

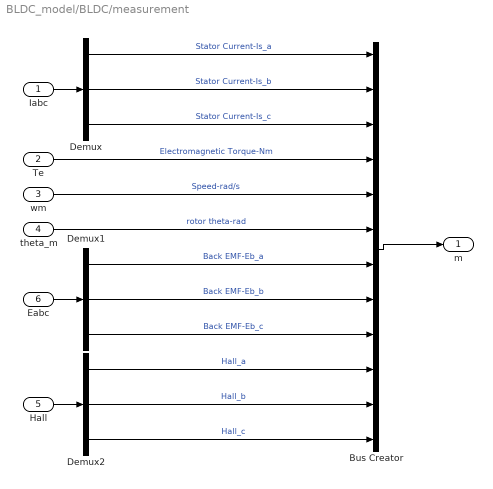
== system BLDC_model/BLDC/measurement ==
  Iabc : Inport
  Te : Inport  Port=2
  wm : Inport  Port=3
  theta_m : Inport  Port=4
  Hall : Inport  Port=5
  Eabc : Inport  Port=6
  Bus Creator : BusCreator  Inputs=12
  Demux : Demux  Outputs=3
  Demux1 : Demux  Outputs=3
  Demux2 : Demux  Outputs=3
  m : Outport
  wires:
  theta_m/1 -> Bus Creator/6  "rotor theta-rad"
  Demux2/3 -> Bus Creator/12  "Hall_c"
  Demux2/2 -> Bus Creator/11  "Hall_b"
  Demux2/1 -> Bus Creator/10  "Hall_a"
  Hall/1 -> Demux2/1
  Demux1/3 -> Bus Creator/9  "Back EMF-Eb_c"
  Demux1/2 -> Bus Creator/8  "Back EMF-Eb_b"
  Demux1/1 -> Bus Creator/7  "Back EMF-Eb_a"
  Eabc/1 -> Demux1/1
  Demux/2 -> Bus Creator/2  "Stator Current-Is_b"
  Bus Creator/1 -> m/1
  wm/1 -> Bus Creator/5  "Speed-rad/s"
  Te/1 -> Bus Creator/4  "Electromagnetic Torque-Nm"
  Demux/3 -> Bus Creator/3  "Stator Current-Is_c"
  Demux/1 -> Bus Creator/1  "Stator Current-Is_a"
  Iabc/1 -> Demux/1

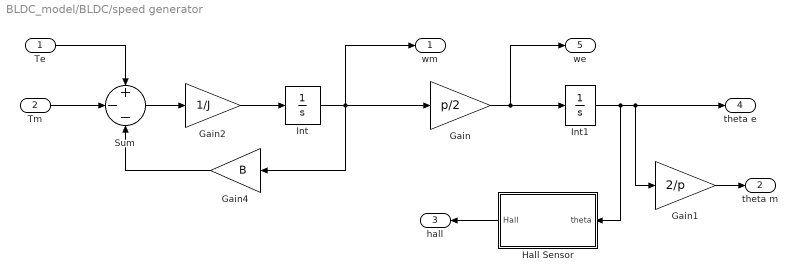
== system BLDC_model/BLDC/speed generator ==
  Te : Inport
  Tm : Inport  Port=2
  Gain : Gain  Gain=p/2  SaturateOnIntegerOverflow=on  OutDataTypeStr=Inherit: Same as input  ParamDataTypeStr=Inherit: Same as input
  Gain1 : Gain  Gain=2/p  SaturateOnIntegerOverflow=on  OutDataTypeStr=Inherit: Same as input  ParamDataTypeStr=Inherit: Same as input
  Gain2 : Gain  Gain=1/J  SaturateOnIntegerOverflow=on  OutDataTypeStr=Inherit: Same as input  ParamDataTypeStr=Inherit: Same as input
  Gain4 : Gain  Gain=B  SaturateOnIntegerOverflow=on  OutDataTypeStr=Inherit: Same as input  ParamDataTypeStr=Inherit: Same as input
  Hall Sensor : Subsystem
  Int : Integrator
  Int1 : Integrator
  Sum : Sum  Inputs=+--  InputSameDT=on  SaturateOnIntegerOverflow=on  OutDataTypeStr=Inherit: Same as first input
  wm : Outport
  theta m : Outport  Port=2
  hall : Outport  Port=3
  theta e : Outport  Port=4
  we : Outport  Port=5
  wires:
  Gain1/1 -> theta m/1
  Hall Sensor/1(Hall) -> hall/1
  Te/1 -> Sum/1
  Tm/1 -> Sum/2
  Gain4/1 -> Sum/3
  Sum/1 -> Gain2/1
  Gain2/1 -> Int/1
  Int/1 -> wm/1, Gain4/1, Gain/1
  Gain/1 -> we/1, Int1/1
  Int1/1 -> Gain1/1, theta e/1, Hall Sensor/1(theta)

== system BLDC_model/BLDC/Back EMF Calculation/Phase a ==
  note: Phi' r
  the,we : Inport
  Demux : Demux  Outputs=2
      settings: DisplayOption=none
  Fcn : Fcn  Expr=cos(u(1))
  Gain4 : Gain  Gain=flux/trap  SaturateOnIntegerOverflow=on  OutDataTypeStr=Inherit: Same as input  ParamDataTypeStr=Inherit: Same as input
  Product1 : Product  SaturateOnIntegerOverflow=on  OutDataTypeStr=Inherit: Same as first input
  Saturation : Saturate  UpperLimit=trap  LowerLimit=-trap
  phi'r : Outport
  E : Outport  Port=2
  wires:
  Fcn/1 -> Saturation/1
  Saturation/1 -> Gain4/1
  Demux/1 -> Fcn/1
  Demux/2 -> Product1/2
  the,we/1 -> Demux/1
  Product1/1 -> E/1
  Gain4/1 -> phi'r/1, Product1/1

== system BLDC_model/BLDC/Back EMF Calculation/Phase b ==
  note: Phi' r
  the,we : Inport
  Demux : Demux  Outputs=2
      settings: DisplayOption=none
  Fcn : Fcn  Expr=cos(u(1)-2*pi/3)
  Gain4 : Gain  Gain=flux/trap  SaturateOnIntegerOverflow=on  OutDataTypeStr=Inherit: Same as input  ParamDataTypeStr=Inherit: Same as input
  Product1 : Product  SaturateOnIntegerOverflow=on  OutDataTypeStr=Inherit: Same as first input
  Saturation : Saturate  UpperLimit=trap  LowerLimit=-trap
  phi'r : Outport
  E : Outport  Port=2
  wires:
  Fcn/1 -> Saturation/1
  Saturation/1 -> Gain4/1
  Gain4/1 -> Product1/1, phi'r/1
  Product1/1 -> E/1
  the,we/1 -> Demux/1
  Demux/2 -> Product1/2
  Demux/1 -> Fcn/1

== system BLDC_model/BLDC/Back EMF Calculation/Phase c ==
  note: Phi' r
  the,we : Inport
  Demux : Demux  Outputs=2
      settings: DisplayOption=none
  Fcn : Fcn  Expr=cos(u(1)+2*pi/3)
  Gain4 : Gain  Gain=flux/trap  SaturateOnIntegerOverflow=on  OutDataTypeStr=Inherit: Same as input  ParamDataTypeStr=Inherit: Same as input
  Product1 : Product  SaturateOnIntegerOverflow=on  OutDataTypeStr=Inherit: Same as first input
  Saturation : Saturate  UpperLimit=trap  LowerLimit=-trap
  phi'r : Outport
  E : Outport  Port=2
  wires:
  Fcn/1 -> Saturation/1
  Saturation/1 -> Gain4/1
  Demux/1 -> Fcn/1
  Demux/2 -> Product1/2
  the,we/1 -> Demux/1
  Product1/1 -> E/1
  Gain4/1 -> phi'r/1, Product1/1

== system BLDC_model/BLDC/Current Calculation/State Ib ==
  Vab,Vbc : Inport
  Eabc : Inport  Port=2
  Fcn : Fcn  Expr=-u(1)+u(2)+u(3)-2*u(4)+u(5)-3*Rs*u(6)
  Gain2 : Gain  Gain=1/(3*Ls)  SaturateOnIntegerOverflow=on  OutDataTypeStr=Inherit: Same as input  ParamDataTypeStr=Inherit: Same as input
  Mux : Mux  Inputs=3
  "s " : Integrator
  Ib : Outport
  wires:
  "s "/1 -> Ib/1, Mux/3
  Fcn/1 -> Gain2/1
  Mux/1 -> Fcn/1
  Eabc/1 -> Mux/2
  Vab,Vbc/1 -> Mux/1
  Gain2/1 -> "s "/1

== system BLDC_model/BLDC/Current Calculation/state Ia ==
  Vab,Vbc : Inport
  Eabc : Inport  Port=2
  Fcn : Fcn  Expr=2*u(1)+u(2)-2*u(3)+u(4)+u(5)-3*Rs*u(6)
  Gain2 : Gain  Gain=1/(3*Ls)  SaturateOnIntegerOverflow=on  OutDataTypeStr=Inherit: Same as input  ParamDataTypeStr=Inherit: Same as input
  Mux : Mux  Inputs=3
  "s " : Integrator
  Ia : Outport
  wires:
  Gain2/1 -> "s "/1
  Vab,Vbc/1 -> Mux/1
  Eabc/1 -> Mux/2
  Mux/1 -> Fcn/1
  Fcn/1 -> Gain2/1
  "s "/1 -> Ia/1, Mux/3

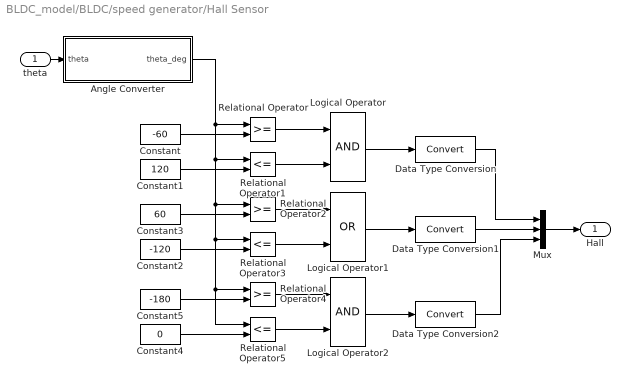
== system BLDC_model/BLDC/speed generator/Hall Sensor ==
  theta : Inport
  Angle Converter : Subsystem
  Constant : Constant  Value=-60
  Constant1 : Constant  Value=120
  Constant2 : Constant  Value=-120
  Constant3 : Constant  Value=60
  Constant4 : Constant  Value=0
  Constant5 : Constant  Value=-180
  Data Type Conversion : DataTypeConversion
  Data Type Conversion1 : DataTypeConversion
  Data Type Conversion2 : DataTypeConversion
  Logical Operator : Logic  AllPortsSameDT=off  OutDataTypeStr=boolean
  Logical Operator1 : Logic  Operator=OR  AllPortsSameDT=off  OutDataTypeStr=boolean
  Logical Operator2 : Logic  AllPortsSameDT=off  OutDataTypeStr=boolean
  Mux : Mux  Inputs=3
  Relational Operator : RelationalOperator  OutDataTypeStr=boolean  RndMeth=Nearest
  Relational Operator1 : RelationalOperator  Operator=<=  OutDataTypeStr=boolean  RndMeth=Nearest
  Relational Operator2 : RelationalOperator  OutDataTypeStr=boolean  RndMeth=Nearest
  Relational Operator3 : RelationalOperator  Operator=<=  OutDataTypeStr=boolean  RndMeth=Nearest
  Relational Operator4 : RelationalOperator  OutDataTypeStr=boolean  RndMeth=Nearest
  Relational Operator5 : RelationalOperator  Operator=<=  OutDataTypeStr=boolean  RndMeth=Nearest
  Hall : Outport
  wires:
  Mux/1 -> Hall/1
  Data Type Conversion2/1 -> Mux/3
  Data Type Conversion1/1 -> Mux/2
  Data Type Conversion/1 -> Mux/1
  Logical Operator/1 -> Data Type Conversion/1
  Logical Operator1/1 -> Data Type Conversion1/1
  Logical Operator2/1 -> Data Type Conversion2/1
  Relational Operator5/1 -> Logical Operator2/2
  Relational Operator4/1 -> Logical Operator2/1
  Relational Operator3/1 -> Logical Operator1/2
  Relational Operator2/1 -> Logical Operator1/1
  Relational Operator1/1 -> Logical Operator/2
  Relational Operator/1 -> Logical Operator/1
  Constant4/1 -> Relational Operator5/2
  Constant5/1 -> Relational Operator4/2
  Constant2/1 -> Relational Operator3/2
  Constant3/1 -> Relational Operator2/2
  Constant1/1 -> Relational Operator1/2
  Constant/1 -> Relational Operator/2
  Angle Converter/1(theta_deg) -> Relational Operator5/1, Relational Operator4/1, Relational Operator3/1, Relational Operator2/1, Relational Operator1/1, Relational Operator/1
  theta/1 -> Angle Converter/1(theta)

== system BLDC_model/BLDC/speed generator/Hall Sensor/Angle Converter ==
  theta : Inport
  Trigonometric Function : Trigonometry
  Trigonometric Function1 : Trigonometry  Operator=cos
  Trigonometric Function2 : Trigonometry  Operator=atan2
  rad2deg : Gain  Gain=180/pi
  theta_deg : Outport
  wires:
  rad2deg/1 -> theta_deg/1
  theta/1 -> Trigonometric Function1/1, Trigonometric Function/1
  Trigonometric Function1/1 -> Trigonometric Function2/2
  Trigonometric Function/1 -> Trigonometric Function2/1
  Trigonometric Function2/1 -> rad2deg/1

== matlab function BLDC_model/Subsystem/MATLAB Function ==
  data: angle input; angle_in_range output
function angle_in_range = wrapAngle(angle)

if angle < 0
    angle_in_range = 2*pi + angle;
else
    angle_in_range = angle;
end

end

== matlab function BLDC_model/MATLAB Function ==
  data: angle input; sector output
function sector = angleToSector(angle)

if(11*pi/6 < angle || angle <= pi/6)
    sector = 1;
elseif(pi/6 < angle && angle <= 3*pi/6)
    sector = 2;
elseif(3*pi/6 < angle && angle <= 5*pi/6)
    sector = 3;
elseif(5*pi/6 < angle && angle <= 7*pi/6)
    sector = 4;
elseif(7*pi/6 < angle && angle <= 9*pi/6)
    sector = 5;
elseif(9*pi/6 < angle && angle <= 11*pi/6)
    sector = 6;
else
    sector = 0;
    
end
